simulink subsystem "GlobalMPController"  (R2022b)
settings: Solver=VariableStepAuto  StartTime=0.0  StopTime=10.0  RelTol=1e-3
model mask{c=0}
  mask prompts: c "standard constants"
settings Model: Creator=is123  LastModifiedBy=is123

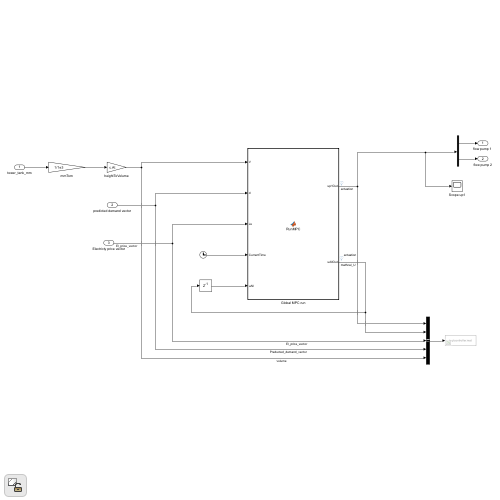
[thumbnail: Simulink's stored preview of the top-level diagram]
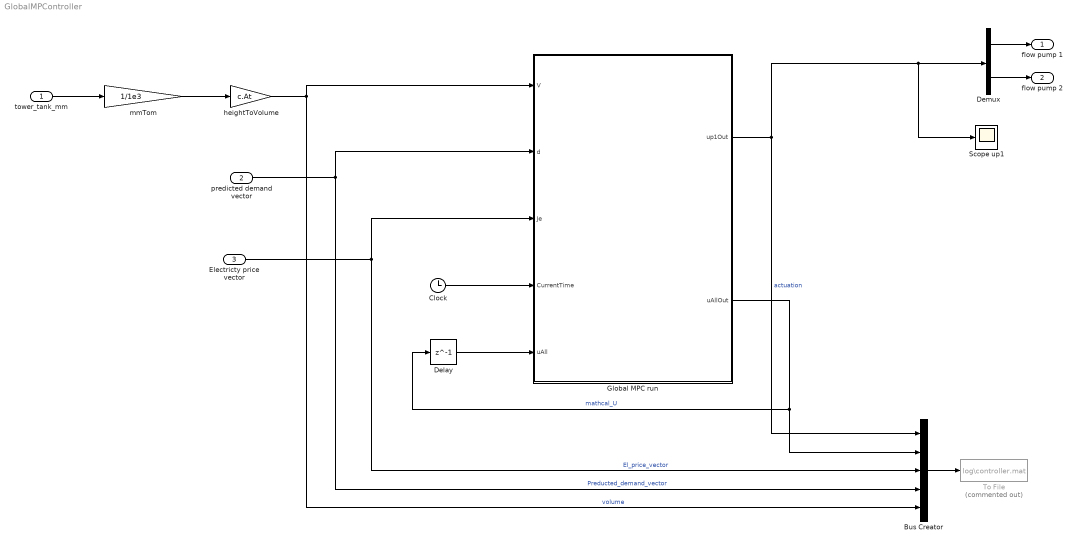
== system GlobalMPController ==
  tower_tank_mm : Inport
  predicted demand vector : Inport  Port=2
  Electricty price vector : Inport  Port=3
  Bus Creator : BusCreator  Inputs=5
  Clock : Clock
  Delay : Delay  DelayLength=1  InitialCondition=zeros(c.Nu*c.Nc,1)
  Demux : Demux  Outputs=2
  Global MPC run : MATLAB Function  TreatAsAtomicUnit=on  SystemSampleTime=3600/c.AccTime
  Scope up1 : Scope
  To File : ToFile  Commented=on  Filename=log\controller.mat  MatrixName=ctrl  SaveFormat=Timeseries
  heightToVolume : Gain  Gain=c.At
  mmTom : Gain  Gain=1/1e3
  "flow pump 1 " : Outport
  flow pump 2 : Outport  Port=2
  wires:
  Global MPC run/1(up1Out) -> Bus Creator/1, Demux/1, Scope up1/1  "actuation"
  Global MPC run/2(uAllOut) -> Delay/1, Bus Creator/2  "mathcal_U"
  Delay/1 -> Global MPC run/5(uAll)
  predicted demand vector/1 -> Global MPC run/2(d), Bus Creator/4  "Preducted_demand_vector"
  Electricty price vector/1 -> Global MPC run/3(Je), Bus Creator/3  "El_price_vector"
  Demux/2 -> flow pump 2/1
  Demux/1 -> "flow pump 1 "/1
  heightToVolume/1 -> Global MPC run/1(V), Bus Creator/5  "volume"
  tower_tank_mm/1 -> mmTom/1
  mmTom/1 -> heightToVolume/1
  Bus Creator/1 -> To File/1
  Clock/1 -> Global MPC run/4(CurrentTime)

== matlab function GlobalMPController/Global MPC run ==
  data: V input; d input; Je input; CurrentTime input; uAll input; up1Out output; uAllOut output
function [up1Out,uAllOut]= RunMPC(V,d, Je,CurrentTime,uAll)
%needed to make the function run 
%coder.extrinsic('mpcRunV2')
coder.extrinsic('mpcRunV2Casadi')


%Loading in standard Constants
c=scaled_standard_constants;

% Scaling the eletricity price if it is desired: 
    if c.scaledEletricityPrice == true
        Je=Je/norm(Je); 
    end 

%Giving the system 10 minuts to start up
if CurrentTime <200 
    up1Out=zeros(c.Nu,1);
    uAllOut=zeros(c.Nu*c.Nc,1);    
else 
    %Need putting the demand, current water volume, and eletricity price into
    %a new struct 
    data.V=V;
    data.d=d;
    data.Je=Je;
    
    %Setting size of the output, neccesary to make Simulink run 
    up1Out=zeros(c.Nu,1);
    uAllOut=zeros(c.Nu*c.Nc,1);
    
    
    
    %solving the global model control problem 
    [up1OutTemp,uAllOutTemp]=mpcRunV2Casadi(data,uAll,c.scaled); 

    %Picking out the outputs: 
    up1Out=up1OutTemp;
    uAllOut=uAllOutTemp;

end 

end
